simulink subsystem "coolantTemp"  (R2022b)
settings: Solver=VariableStepAuto  StartTime=0.0  StopTime=10.0  RelTol=1e-3
libraries: cooling_lib x3, Raptor_lib x3
settings Model: Creator=serga  LastModifiedBy=serga

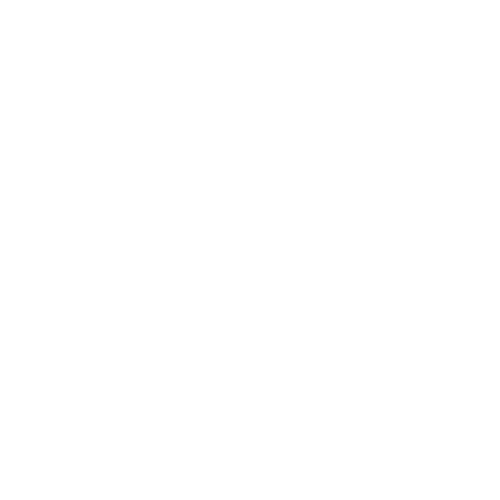
[thumbnail: Simulink's stored preview of the top-level diagram]
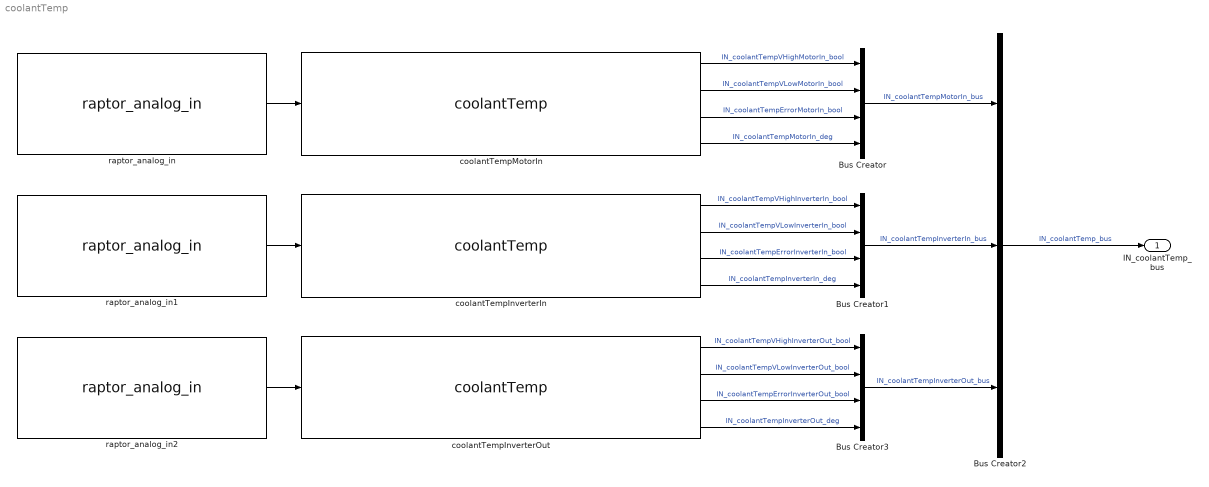
== system coolantTemp ==
  Bus Creator : BusCreator  Inputs=4
  Bus Creator1 : BusCreator  Inputs=4
  Bus Creator2 : BusCreator  Inputs=3
  Bus Creator3 : BusCreator  Inputs=4
  coolantTempInverterIn : cooling_lib/coolantTemp  pos='InverterIn'
  coolantTempInverterOut : cooling_lib/coolantTemp  pos='InverterOut'
  coolantTempMotorIn : cooling_lib/coolantTemp  pos='MotorIn'
  raptor_analog_in : Raptor_lib/Input & Output/raptor_analog_in  resourceValues=INPUT2|INPUT3|INPUT4|INPUT5|INPUT6|INPUT7|INPUT8|INPUT9|INPUT10|INPUT11|INPUT12|INPUT13|INPUT14|INPUT15|INPUT16|INPUT17|INPUT18|INPUT19|INPUT20|INPUT21|INPUT22|INPUT23|INPUT24|INPUT25|INPUT26|INPUT27|INPUT28|INPUT29|INPUT30|INPUT31|INPUT32|(None)  resource=INPUT10  rangeValues=0 - 5 V  range=0 - 5 V  filterrateValues=[]  filterrate='RAPTOR MASK DEFAULT'  resolutionValues=[]  resolution=[]  pullUDValues=681k PU  pullUD=681k PU
      settings: SourceProductName=Raptor
  raptor_analog_in1 : Raptor_lib/Input & Output/raptor_analog_in  resourceValues=INPUT2|INPUT3|INPUT4|INPUT5|INPUT6|INPUT7|INPUT8|INPUT9|INPUT10|INPUT11|INPUT12|INPUT13|INPUT14|INPUT15|INPUT16|INPUT17|INPUT18|INPUT19|INPUT20|INPUT21|INPUT22|INPUT23|INPUT24|INPUT25|INPUT26|INPUT27|INPUT28|INPUT29|INPUT30|INPUT31|INPUT32|(None)  resource=INPUT11  rangeValues=0 - 5 V  range=0 - 5 V  filterrateValues=[]  filterrate='RAPTOR MASK DEFAULT'  resolutionValues=[]  resolution=[]  pullUDValues=681k PU  pullUD=681k PU
      settings: SourceProductName=Raptor
  raptor_analog_in2 : Raptor_lib/Input & Output/raptor_analog_in  resourceValues=INPUT2|INPUT3|INPUT4|INPUT5|INPUT6|INPUT7|INPUT8|INPUT9|INPUT10|INPUT11|INPUT12|INPUT13|INPUT14|INPUT15|INPUT16|INPUT17|INPUT18|INPUT19|INPUT20|INPUT21|INPUT22|INPUT23|INPUT24|INPUT25|INPUT26|INPUT27|INPUT28|INPUT29|INPUT30|INPUT31|INPUT32|(None)  resource=INPUT12  rangeValues=0 - 5 V  range=0 - 5 V  filterrateValues=[]  filterrate='RAPTOR MASK DEFAULT'  resolutionValues=[]  resolution=[]  pullUDValues=422k PD  pullUD=422k PD
      settings: SourceProductName=Raptor
  IN_coolantTemp_bus : Outport
  wires:
  coolantTempMotorIn/1 -> Bus Creator/1  "IN_coolantTempVHighMotorIn_bool"
  coolantTempMotorIn/2 -> Bus Creator/2  "IN_coolantTempVLowMotorIn_bool"
  coolantTempMotorIn/3 -> Bus Creator/3  "IN_coolantTempErrorMotorIn_bool"
  coolantTempMotorIn/4 -> Bus Creator/4  "IN_coolantTempMotorIn_deg"
  coolantTempInverterIn/1 -> Bus Creator1/1  "IN_coolantTempVHighInverterIn_bool"
  coolantTempInverterIn/2 -> Bus Creator1/2  "IN_coolantTempVLowInverterIn_bool"
  coolantTempInverterIn/3 -> Bus Creator1/3  "IN_coolantTempErrorInverterIn_bool"
  coolantTempInverterIn/4 -> Bus Creator1/4  "IN_coolantTempInverterIn_deg"
  Bus Creator1/1 -> Bus Creator2/2  "IN_coolantTempInverterIn_bus"
  Bus Creator/1 -> Bus Creator2/1  "IN_coolantTempMotorIn_bus"
  Bus Creator2/1 -> IN_coolantTemp_bus/1  "IN_coolantTemp_bus"
  Bus Creator3/1 -> Bus Creator2/3  "IN_coolantTempInverterOut_bus"
  coolantTempInverterOut/1 -> Bus Creator3/1  "IN_coolantTempVHighInverterOut_bool"
  coolantTempInverterOut/2 -> Bus Creator3/2  "IN_coolantTempVLowInverterOut_bool"
  coolantTempInverterOut/3 -> Bus Creator3/3  "IN_coolantTempErrorInverterOut_bool"
  coolantTempInverterOut/4 -> Bus Creator3/4  "IN_coolantTempInverterOut_deg"
  raptor_analog_in/1 -> coolantTempMotorIn/1
  raptor_analog_in1/1 -> coolantTempInverterIn/1
  raptor_analog_in2/1 -> coolantTempInverterOut/1
